simulink model "Modulate"  (R2024a)
settings: Solver=VariableStepAuto  StartTime=0.0  StopTime=10.0  RelTol=1e-3
libraries: spsTriangleGeneratorLib x2, sps_lib x1
settings Model: Creator=50803  LastModifiedBy=50803

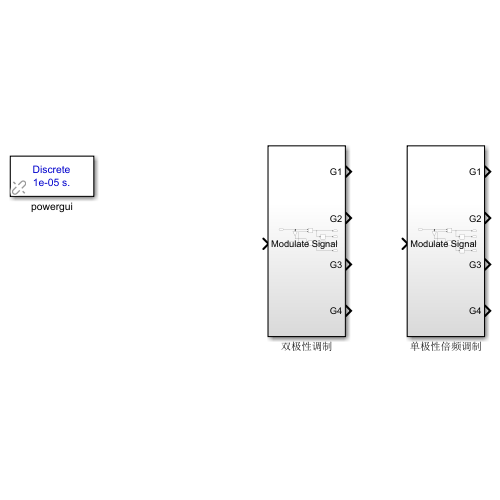
[thumbnail: Simulink's stored preview of the top-level diagram]
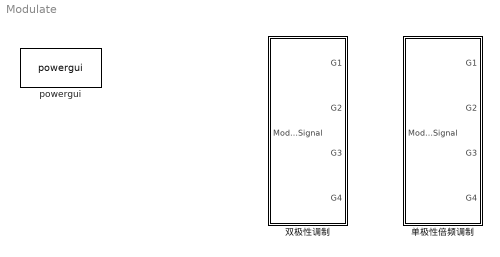
== system Modulate ==
  powergui : sps_lib/powergui  Priority=1  SimulationMode=Discrete  SampleTime=1E-5  frequency=60  Iterations=50  frequencyindice=0  Pbase=100e6  ErrMax=1e-4  UnitsV=kV  UnitsW=MW  buscounter=0  FunctionMessages=off  echomessages=off  EnableUseOfTLC=off  CurrentSourceSwitches=off  DisableSnubberDevices=off  DisableRonSwitches=off  DisableVfSwitches=off  DisplayEquations=off  AutomaticDiscreteSolvers=off  SolverType=Tustin/Backward Euler (TBE)  Interpol=off  ExternalGateDelay=off  methode=off  Ts=100  x0status=blocks  SPID=on  SwTol=0  HookPort=off  NonlinearTolerance=1e-4  nMaxIteration=100  ContinueOnMaxIteration=off  RestoreLinks=warning  ResistiveCurrentMeasurement=off  Frange=[0:2:500]  Ylog=off  Xlog=on  ShowGrid=off  save=off  variable=ZData  structure=0  ZoomFFT=off  StartTime=0.0  cycles=1  DisplayStyle=1  fundamental=60  FreqAxis=off  MaxFrequency=1000  frequencyindicesteady=1  RmsSteady=1  display=off
  单极性倍频调制 : Subsystem
  双极性调制 : Subsystem

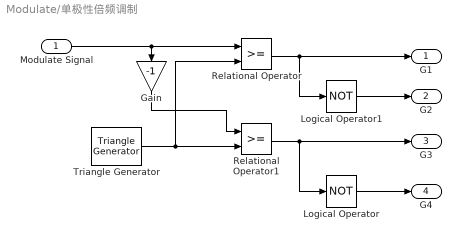
== system Modulate/单极性倍频调制 ==
  Modulate Signal : Inport
  Gain : Gain  Gain=-1
  Logical Operator : Logic  Operator=NOT  AllPortsSameDT=off  OutDataTypeStr=boolean
  Logical Operator1 : Logic  Operator=NOT  AllPortsSameDT=off  OutDataTypeStr=boolean
  Relational Operator : RelationalOperator  OutDataTypeStr=boolean  RndMeth=Simplest  InputSameDT=off
  Relational Operator1 : RelationalOperator  OutDataTypeStr=boolean  RndMeth=Simplest  InputSameDT=off
  Triangle Generator : spsTriangleGeneratorLib/Triangle Generator  Freq=20*1e3  Phase=180  Ts=0
  G1 : Outport
  G2 : Outport  Port=2
  G3 : Outport  Port=3
  G4 : Outport  Port=4
  wires:
  Logical Operator1/1 -> G2/1
  Relational Operator/1 -> Logical Operator1/1, G1/1
  Triangle Generator/1 -> Relational Operator1/2, Relational Operator/2
  Relational Operator1/1 -> Logical Operator/1, G3/1
  Modulate Signal/1 -> Relational Operator/1, Gain/1
  Gain/1 -> Relational Operator1/1
  Logical Operator/1 -> G4/1

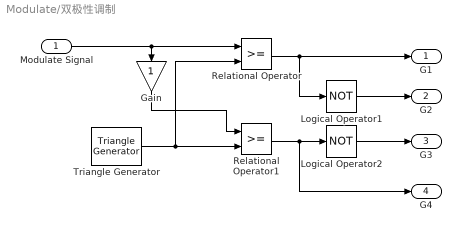
== system Modulate/双极性调制 ==
  Modulate Signal : Inport
  Gain : Gain
  Logical Operator1 : Logic  Operator=NOT  AllPortsSameDT=off  OutDataTypeStr=boolean
  Logical Operator2 : Logic  Operator=NOT  AllPortsSameDT=off  OutDataTypeStr=boolean
  Relational Operator : RelationalOperator  OutDataTypeStr=boolean  RndMeth=Simplest  InputSameDT=off
  Relational Operator1 : RelationalOperator  OutDataTypeStr=boolean  RndMeth=Simplest  InputSameDT=off
  Triangle Generator : spsTriangleGeneratorLib/Triangle Generator  Freq=20*1e3  Phase=180  Ts=0
  G1 : Outport
  G2 : Outport  Port=2
  G3 : Outport  Port=3
  G4 : Outport  Port=4
  wires:
  Relational Operator1/1 -> G4/1, Logical Operator2/1
  Gain/1 -> Relational Operator1/1
  Modulate Signal/1 -> Gain/1, Relational Operator/1
  Triangle Generator/1 -> Relational Operator/2, Relational Operator1/2
  Relational Operator/1 -> G1/1, Logical Operator1/1
  Logical Operator1/1 -> G2/1
  Logical Operator2/1 -> G3/1
